simulink model "IQinputToy"  (R2016b)
settings: Solver=ode45  StartTime=0.0  StopTime=5e-6  MaxStep=1e-6  RelTol=1e-3  EnableMultiTasking=on
libraries: xbsIndex_r4 x6
settings Model: Creator=ssmith  LastModifiedBy=ssmith
settings DataIOCC: LimitDataPoints=on  SaveFormat=Array
settings OptimizationCC: LifeSpan=inf
settings DebuggingCC: UnderspecifiedInitializationDetection=Classic  MergeDetectMultiDrivingBlocksExec=none  SolverPrmCheckMsg=warning  SFUnexpectedBacktrackingDiag=warning  SFNoUnconditionalDefaultTransitionDiag=warning  SFExecutionAtInitializationDiag=none
settings HardwareCC: ProdBitPerPointer=32  ProdBitPerSizeT=32  ProdBitPerPtrDiffT=32  ProdLargestAtomicFloat=None  ProdIntDivRoundTo=Undefined  ProdEndianess=Unspecified  ProdWordSize=32  ProdHWDeviceType=32-bit Generic
settings ModelReferenceCC: PropagateSignalLabelsOutOfModel=off
settings GRTTargetCC: TargetLangStandard=C89/C90 (ANSI)  GeneratePreprocessorConditionals=Disable all
settings ConfigComp: CovMetricSettings=dw  CovHtmlReporting=on  CovSaveCumulativeToWorkspaceVar=on  CovSaveSingleToWorkspaceVar=on  CovExternalEMLEnable=off  CovSFcnEnable=off

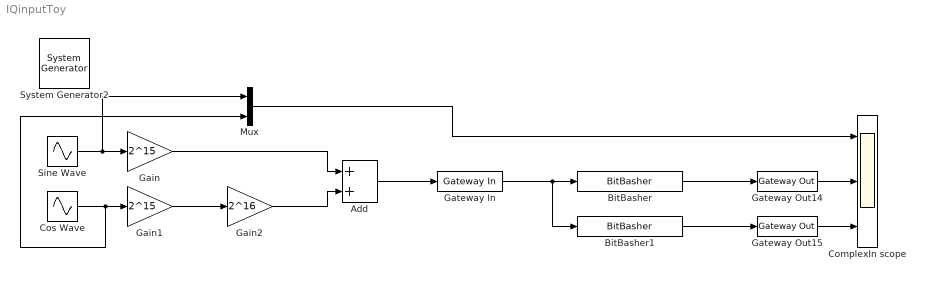
== system IQinputToy ==
  " System Generator2" : xbsIndex_r4/ System Generator  Tag=genX  xilinxfamily=kintex7  part=xc7k70t  speed=-1  package=fbg484  synthesis_tool=Vivado  clock_wrapper=Clock Enables  directory=./netlist  proj_type=Vivado  Synth_file=Vivado Synthesis Defaults  Impl_file=Vivado Implementation Defaults  testbench=off  simulink_period=10e-9  sysclk_period=10  dcm_input_clock_period=10  incr_netlist=off  trim_vbits=Everywhere in SubSystem  dbl_ovrd=According to Block Masks  core_generation=According to Block Masks  run_coregen=off  deprecated_control=off  eval_field=0  block_type=sysgen
  Add : Sum  RndMeth=Nearest
  BitBasher : xbsIndex_r4/BitBasher  bitexpr=hi = {in[31:16]}  display_expr=on  sr_1=hi  arith_type1="Signed  (2's comp)"  bin_pt1=15  sr_2=2  arith_type2=Unsigned  bin_pt2=0  sr_3=3  arith_type3=Unsigned  bin_pt3=0  sr_4=4  arith_type4=Unsigned  bin_pt4=0  dbl_ovrd=off  block_type=bitbasher
  BitBasher1 : xbsIndex_r4/BitBasher  bitexpr=lo = {in[15:0]}  display_expr=on  sr_1=lo  arith_type1="Signed  (2's comp)"  bin_pt1=15  sr_2=2  arith_type2=Unsigned  bin_pt2=0  sr_3=3  arith_type3=Unsigned  bin_pt3=0  sr_4=4  arith_type4=Unsigned  bin_pt4=0  dbl_ovrd=off  block_type=bitbasher
  ComplexIn scope : Scope  NumInputPorts=3
  Cos Wave : Sin  Amplitude=0.999  Frequency=2*pi*1e6 * 2  Phase=pi/2  SampleTime=0
  Gain : Gain  Gain=2^15  OutDataTypeStr=uint16  RndMeth=Nearest
  Gain1 : Gain  Gain=2^15  OutDataTypeStr=int16  RndMeth=Nearest
  Gain2 : Gain  Gain=2^16  OutDataTypeStr=uint32  RndMeth=Nearest
  Gateway In : xbsIndex_r4/Gateway In  gui_display_data_type=Fixed-point  arith_type=Unsigned  n_bits=32  bin_pt=0  preci_type=Single  exp_width=8  frac_width=24  rows=1  columns=1  quantization="Round  (unbiased: +/- Inf)"  overflow=Saturate  period=10e-9  UseAsADC=off  ADCChannel='1'  interface=None  automatic_assignment=on  address_offset=hex2dec('00')  intf_name=''  intf_description=''  default_value=0  timing_constraint=None  locs_specified=off  LOCs={}  io_standard={}  inherit_from_input=off  hdl_port=on  dbl_ovrd=off  block_type=gatewayin
  Gateway Out14 : xbsIndex_r4/Gateway Out  inherit_from_input=off  hdl_port=off  rows=1  columns=1  UseAsDAC=off  DACChannel='1'  interface=None  automatic_assignment=on  address_offset=hex2dec('00')  intf_name=''  intf_description=''  timing_constraint=None  locs_specified=off  LOCs={}  io_standard={}  block_type=gatewayout
  Gateway Out15 : xbsIndex_r4/Gateway Out  inherit_from_input=off  hdl_port=off  rows=1  columns=1  UseAsDAC=off  DACChannel='1'  interface=None  automatic_assignment=on  address_offset=hex2dec('00')  intf_name=''  intf_description=''  timing_constraint=None  locs_specified=off  LOCs={}  io_standard={}  block_type=gatewayout
  Mux : Mux  Inputs=2
  Sine Wave : Sin  Amplitude=0.999  Frequency=2*pi*1e6  SampleTime=0
  wires:
  Gateway Out15/1 -> ComplexIn scope/3
  Add/1 -> Gateway In/1
  Gateway Out14/1 -> ComplexIn scope/2
  Gateway In/1 -> BitBasher1/1, BitBasher/1
  BitBasher/1 -> Gateway Out14/1
  BitBasher1/1 -> Gateway Out15/1
  Gain1/1 -> Gain2/1
  Cos Wave/1 -> Mux/2, Gain1/1
  Sine Wave/1 -> Mux/1, Gain/1
  Mux/1 -> ComplexIn scope/1
  Gain/1 -> Add/1
  Gain2/1 -> Add/2
